simulink model "Pt_Engine_CS8"  (Simulink 7.0)
settings: Solver=ode45  StartTime=0  StopTime=20  FixedStep=TSTEP  RelTol=1e-3
PreLoadFcn:
  | cd Extensions/Simulink/pt_engine
  | mengine_carpet_eclass
  | Run_ft4wd_eclass
  | cd ../../..
undefined symbols (not defined in the file): AV_ENG_IDLE, IENG, ITC_INPUT_SHAFT, MENGINE_CARPET
libraries: Solver_SF x1
settings Model: Creator=dhall  LastModifiedBy=ywata  ExtModeTrigMode=oneshot  ExtModeArmWhenConnect=off
settings DataIOCC: LimitDataPoints=off  SaveOutput=off  SaveTime=off  SignalLoggingName=sigsOut
settings OptimizationCC: BooleanDataType=off
settings DebuggingCC: SaveWithParameterizedLinksMsg=none  SignalResolutionControl=TryResolveAllWithWarning  SolverPrmCheckMsg=none  MultiTaskDSMMsg=warning  MultiTaskCondExecSysMsg=none  StrictBusMsg=None
settings HardwareCC: TargetUnknown=on
settings RTWCC: IncludeERTFirstTime=on
settings GRTTargetCC: TargetFcnLib=ansi_tfl_tmw.mat  ModelReferenceCompliant=off  MatFileLogging=off

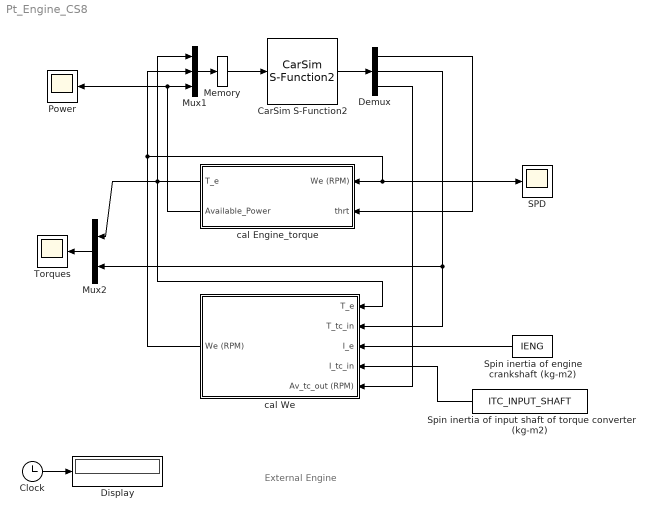
== system Pt_Engine_CS8 ==
  note: External Engine
  CarSim S-Function2 : Solver_SF/CarSim S-Function2  Priority=1  VehicleCode=???
      settings: AttributesFormatString=Vehicle Code: %<VehicleCode>
  Clock : Clock
      settings: Decimation=10
  Demux : Demux  Outputs=3
  Display : Display
  Memory : Memory
  Mux1 : Mux  Inputs=3
  Mux2 : Mux  Orientation=left  Inputs=2
  Power : Scope
      settings: TimeRange=20  YMin=0  YMax=250
  SPD : Scope
      settings: TimeRange=20  YMin=500  YMax=4500
  Spin inertia of engine crankshaft (kg-m2) : Constant  Orientation=left  Value=IENG  OutDataType=sfix(16)  OutScaling=2^0
  Spin inertia of input shaft of torque converter (kg-m2) : Constant  Orientation=left  Value=ITC_INPUT_SHAFT  OutDataType=sfix(16)  OutScaling=2^0
  Torques : Scope
      settings: TimeRange=20  YMin=-50  YMax=600
  cal Engine_torque : Subsystem  Orientation=left
  cal We : Subsystem  Orientation=left
  wires:
  cal We/1(We (RPM)) -> cal Engine_torque/1(We (RPM)), SPD/1, Mux1/2
  Spin inertia of engine crankshaft (kg-m2)/1 -> cal We/3(I_e)
  Spin inertia of input shaft of torque converter (kg-m2)/1 -> cal We/4(I_tc_in)
  cal Engine_torque/1(T_e) -> Mux2/1, cal We/1(T_e), Mux1/1
  CarSim S-Function2/1 -> Demux/1
  Demux/1 -> cal Engine_torque/2(thrt)
  Demux/2 -> cal We/2(T_tc_in), Mux2/2
  Mux2/1 -> Torques/1
  Clock/1 -> Display/1
  cal Engine_torque/2(Available_Power) -> Power/1, Mux1/3
  Demux/3 -> cal We/5(Av_tc_out (RPM))
  Mux1/1 -> Memory/1
  Memory/1 -> CarSim S-Function2/1

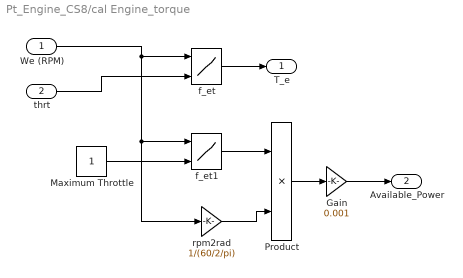
== system Pt_Engine_CS8/cal Engine_torque ==
  We (RPM) : Inport  OutDataType=sfix(16)  OutScaling=2^0
  thrt : Inport  Port=2  OutDataType=sfix(16)  OutScaling=2^0
  Gain : Gain  Gain=0.001  ParameterDataType=sfix(16)  ParameterScaling=2^0  OutDataType=sfix(16)  OutScaling=2^0  SaturateOnIntegerOverflow=on
  Maximum Throttle : Constant  OutDataType=sfix(16)  OutScaling=2^0
  Product : Product  OutDataType=sfix(16)  OutScaling=2^0  SaturateOnIntegerOverflow=on  InputSameDT=on
  f_et : Lookup2D  RowIndex=MENGINE_CARPET(2:19,1)  ColumnIndex=MENGINE_CARPET(1,2:11)  Table=MENGINE_CARPET(2:19,2:11)  OutDataType=sfix(16)  OutScaling=2^0  SaturateOnIntegerOverflow=on  InputSameDT=on
  f_et1 : Lookup2D  RowIndex=MENGINE_CARPET(2:19,1)  ColumnIndex=MENGINE_CARPET(1,2:11)  Table=MENGINE_CARPET(2:19,2:11)  OutDataType=sfix(16)  OutScaling=2^0  SaturateOnIntegerOverflow=on  InputSameDT=on
  rpm2rad : Gain  Gain=1/(60/2/pi)  ParameterDataType=sfix(16)  ParameterScaling=2^0  OutDataType=sfix(16)  OutScaling=2^0  SaturateOnIntegerOverflow=on
  T_e : Outport
  Available_Power : Outport  Port=2
  wires:
  We (RPM)/1 -> f_et/1, f_et1/1, rpm2rad/1
  f_et/1 -> T_e/1
  thrt/1 -> f_et/2
  Maximum Throttle/1 -> f_et1/2
  f_et1/1 -> Product/1
  rpm2rad/1 -> Product/2
  Product/1 -> Gain/1
  Gain/1 -> Available_Power/1

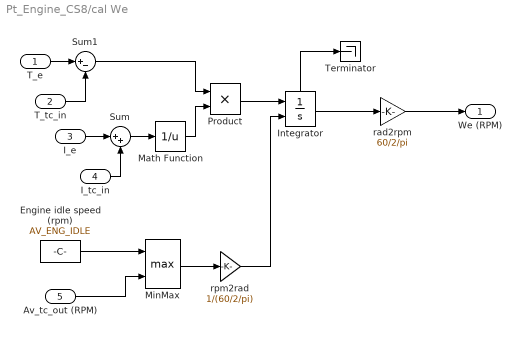
== system Pt_Engine_CS8/cal We ==
  T_e : Inport  OutDataType=sfix(16)  OutScaling=2^0
  T_tc_in : Inport  Port=2  OutDataType=sfix(16)  OutScaling=2^0
  I_e : Inport  Port=3  OutDataType=sfix(16)  OutScaling=2^0
  I_tc_in : Inport  Port=4  OutDataType=sfix(16)  OutScaling=2^0
  Av_tc_out (RPM) : Inport  Port=5  OutDataType=sfix(16)  OutScaling=2^0
  Engine idle speed (rpm) : Constant  Value=AV_ENG_IDLE  OutDataType=sfix(16)  OutScaling=2^0
  Integrator : Integrator  InitialConditionSource=external  InitialCondition=AV_ENG_IDLE*2*pi/60  ShowStatePort=on
  Math Function : Math  Operator=reciprocal  SaturateOnIntegerOverflow=on
  MinMax : MinMax  Function=max  Inputs=2  SaturateOnIntegerOverflow=on  InputSameDT=on
  Product : Product  OutDataType=sfix(16)  OutScaling=2^0  SaturateOnIntegerOverflow=on  InputSameDT=on
  Sum : Sum  Inputs=|++  OutDataType=sfix(16)  OutScaling=2^0  SaturateOnIntegerOverflow=on  InputSameDT=on
  Sum1 : Sum  Inputs=|+-  OutDataType=sfix(16)  OutScaling=2^0  SaturateOnIntegerOverflow=on  InputSameDT=on
  Terminator : Terminator
  rad2rpm : Gain  Gain=60/2/pi  ParameterDataType=sfix(16)  ParameterScaling=2^0  OutDataType=sfix(16)  OutScaling=2^0  SaturateOnIntegerOverflow=on
  rpm2rad : Gain  Gain=1/(60/2/pi)  ParameterDataType=sfix(16)  ParameterScaling=2^0  OutDataType=sfix(16)  OutScaling=2^0  SaturateOnIntegerOverflow=on
  We (RPM) : Outport
  wires:
  rpm2rad/1 -> Integrator/2
  Integrator/1 -> rad2rpm/1
  Product/1 -> Integrator/1
  I_tc_in/1 -> Sum/2
  I_e/1 -> Sum/1
  T_tc_in/1 -> Sum1/2
  Sum/1 -> Math Function/1
  T_e/1 -> Sum1/1
  Sum1/1 -> Product/1
  Math Function/1 -> Product/2
  rad2rpm/1 -> We (RPM)/1
  Engine idle speed (rpm)/1 -> MinMax/1
  Av_tc_out (RPM)/1 -> MinMax/2
  MinMax/1 -> rpm2rad/1
  Integrator/State -> Terminator/1
